simulink model "testSubSystemMIMO"  (Simulink 7.4)
settings: Solver=ode45  StartTime=0.0  StopTime=10.0  MaxStep=0.01  RelTol=1e-3
libraries: BLOM_Lib x2
settings Model: Creator=JJK  LastModifiedBy=JJK
settings DebuggingCC: SolverPrmCheckMsg=none

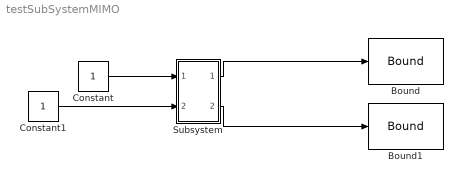
== system testSubSystemMIMO ==
  Bound : BLOM_Lib/Bound  SystemSampleTime=-1  ub=inf  lb=-inf  initial_step=on  final_step=on  intermediate_step=on
  Bound1 : BLOM_Lib/Bound  SystemSampleTime=-1  ub=inf  lb=-inf  initial_step=on  final_step=on  intermediate_step=on
  Constant : Constant  OutDataType=fixdt(1, 16)  OutScaling=2^0
  Constant1 : Constant  OutDataType=fixdt(1, 16)  OutScaling=2^0
  Subsystem : Subsystem
  wires:
  Constant/1 -> Subsystem/1(In1)
  Subsystem/1(Out1) -> Bound/1
  Constant1/1 -> Subsystem/2(In2)
  Subsystem/2(Out2) -> Bound1/1

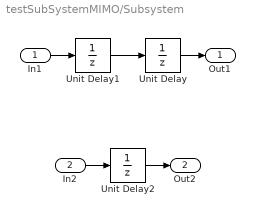
== system testSubSystemMIMO/Subsystem ==
  In1 : Inport
  In2 : Inport  Port=2
  Unit Delay : UnitDelay  SampleTime=-1
  Unit Delay1 : UnitDelay  SampleTime=-1
  Unit Delay2 : UnitDelay  SampleTime=-1
  Out1 : Outport
  Out2 : Outport  Port=2
  wires:
  Unit Delay1/1 -> Unit Delay/1
  Unit Delay/1 -> Out1/1
  In1/1 -> Unit Delay1/1
  In2/1 -> Unit Delay2/1
  Unit Delay2/1 -> Out2/1
